simulink model "AHRS_Voter_Harness_HLR_13"  (R2025a)
settings: Solver=FixedStepDiscrete  StartTime=0.0  StopTime=10.0  RelTol=1e-3  EnableMultiTasking=on
Description:
  | Test harness for HLR_13.
settings Model: DataDictionary=DD_AHRS_Voter.sldd  EnableAccessToBaseWorkspace=off  Creator=The MathWorks, Inc.  LastModifiedBy=The MathWorks, Inc.
settings SolverCC: AlgebraicLoopSolver=TrustRegion  MaxZcPerStep=1.0
settings DataIOCC: LimitDataPoints=on
settings OptimizationCC: BlockReduction=off  DefaultParameterBehavior=Inlined  UseDivisionForNetSlopeComputation=on  UseFloatMulNetSlope=on  InlineInvariantSignals=on  EnhancedBackFolding=on  PassReuseOutputArgsAs=Individual arguments  EfficientFloat2IntCast=on  EfficientMapNaN2IntZero=off  LifeSpan=inf  MaxStackSize=inf  OptimizeBlockOrder=speed  EfficientTunableParamExpr=on
settings DebuggingCC: SignalInfNanChecking=error  SignalRangeChecking=error  ReadBeforeWriteMsg=EnableAllAsError  WriteAfterWriteMsg=EnableAllAsError  WriteAfterReadMsg=EnableAllAsError  AlgebraicLoopMsg=error  ArtificialAlgebraicLoopMsg=error  SaveWithDisabledLinksMsg=error  SaveWithParameterizedLinksMsg=error  BlockPriorityViolationMsg=error  SolverPrmCheckMsg=error  InheritedTsInSrcMsg=error  SingleTaskRateTransMsg=error  TasksWithSamePriorityMsg=error  SigSpecEnsureSampleTimeMsg=error  CheckMatrixSingularityMsg=error  IntegerOverflowMsg=error  ParameterUnderflowMsg=error  ParameterPrecisionLossMsg=error  ParameterTunabilityLossMsg=error  UnderSpecifiedDataTypeMsg=error  UnnecessaryDatatypeConvMsg=warning  VectorMatrixConversionMsg=error  SignalLabelMismatchMsg=error  UnconnectedInputMsg=error  UnconnectedOutputMsg=error  UnconnectedLineMsg=error  SFcnCompatibilityMsg=error  UniqueDataStoreMsg=error  BusObjectLabelMismatch=error  RootOutportRequireBusObject=error  AssertControl=DisableAll  AllowSymbolicDim=off  ModelReferenceIOMismatchMessage=error  UnknownTsInhSupMsg=error  ModelReferenceDataLoggingMessage=error  ModelReferenceSymbolNameMessage=none  StateNameClashWarn=warning  PregeneratedLibrarySubsystemCodeDiagnostic=none  StrictBusMsg=ErrorOnBusTreatedAsVector  NonBusSignalsTreatedAsBus=error  SFInvalidInputDataAccessInChartInitDiag=error  SFTransitionOutsideNaturalParentDiag=error  SFUnreachableExecutionPathDiag=error  SFUndirectedBroadcastEventsDiag=error  SFTransitionActionBeforeConditionDiag=error  SFExecutionAtInitializationDiag=none  IntegerSaturationMsg=error  ArithmeticOperatorsInVariantConditions=warning
settings HardwareCC: ProdBitPerPointer=32.0  ProdBitPerSizeT=32.0  ProdBitPerPtrDiffT=32.0  ProdLargestAtomicInteger=Long  ProdWordSize=32.0  ProdHWDeviceType=ARM Compatible->ARM 10
settings ModelReferenceCC: EnableRefExpFcnMdlSchedulingChecks=on  ModelReferenceNumInstancesAllowed=Single  PropagateSignalLabelsOutOfModel=off
settings SFSimCC: CompileTimeRecursionLimit=0.0  EnableRuntimeRecursion=off  MATLABDynamicMemAlloc=off  CustomCodeUndefinedFunction=UseInterfaceOnly
settings RTWCC: SystemTargetFile=ert.tlc  GenCodeOnly=on  TemplateMakefile=ert_default_tmf  GenerateReport=on  BuildConfiguration=Faster Runs  IncludeHyperlinkInReport=on  LaunchReport=on  GenerateTraceInfo=on  GenerateTraceReport=on  GenerateTraceReportSl=on  GenerateTraceReportSf=on  GenerateTraceReportEml=on  GenerateCodeMetricsReport=on  GPUComputeCapability=3.5  DLArmComputeVersion=19.05  Description=Embedded Coder
settings CodeAppCC: ForceParamTrailComments=on  IgnoreCustomStorageClasses=off  MATLABFcnDesc=on  MangleLength=4.0  StateflowObjectComments=on  ReqsInCode=on
settings ERTTargetCC: ExtModeTransport=0.0  ExtModeStaticAlloc=off  ExtModeMexFile=ext_comm  ExtModeIntrfLevel=Level1  ERTCustomFileTemplate=example_file_process.tlc  PreserveExpressionOrder=on  PreserveIfCondition=on  SuppressUnreachableDefaultCases=off  EnableSignedLeftShifts=off  EnableSignedRightShifts=off  DynamicArrayContainerType=coder::array  TargetLangStandard=C99 (ISO)  UtilityFuncGeneration=Shared location  GenerateSampleERTMain=on  IncludeMdlTerminateFcn=off  SuppressErrorStatus=on  SupportAbsoluteTime=off  SubcomponentCodeInterfacePackaging=Nonreusable function  SupportNonFinite=off  RemoveDisableFunc=on  ParenthesesLevel=Maximum  CastingMode=Standards  GenerateSharedConstants=off

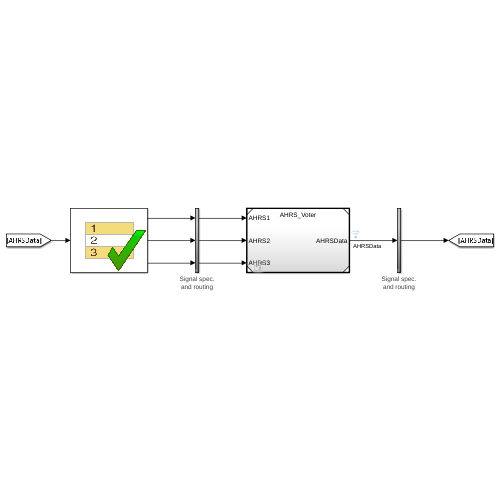
[thumbnail: Simulink's stored preview of the top-level diagram]
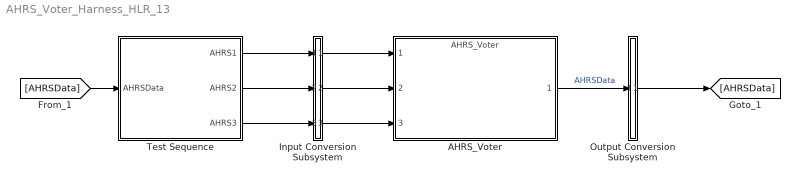
== system AHRS_Voter_Harness_HLR_13 ==
  AHRS_Voter : ModelReference  ModelNameDialog=AHRS_Voter  SimulationMode=Normal  ModelReferenceVersion=3.0
  Input Conversion Subsystem : Subsystem  Tag=__SLT_ICS__  Description=|
      | Signal spec.
      | and routing
      settings: AttributesFormatString=%<Description>
  Output Conversion Subsystem : Subsystem  Tag=__SLT_OCS__  Description=|
      | Signal spec.
      | and routing
      settings: AttributesFormatString=%<Description>
  Test Sequence : Test Sequence  TreatAsAtomicUnit=on
  wires:
  Test Sequence/1(AHRS1) -> Input Conversion Subsystem/1(Inport_1)
  Test Sequence/2(AHRS2) -> Input Conversion Subsystem/2(Inport_2)
  Test Sequence/3(AHRS3) -> Input Conversion Subsystem/3(Inport_3)
  [AHRSData] -> Test Sequence/1(AHRSData)
  Output Conversion Subsystem/1(Outport_1) -> [AHRSData]
  Input Conversion Subsystem/1(Outport_1) -> AHRS_Voter/1
  Input Conversion Subsystem/2(Outport_2) -> AHRS_Voter/2
  Input Conversion Subsystem/3(Outport_3) -> AHRS_Voter/3
  AHRS_Voter/1 -> Output Conversion Subsystem/1(Inport_1)  "AHRSData"

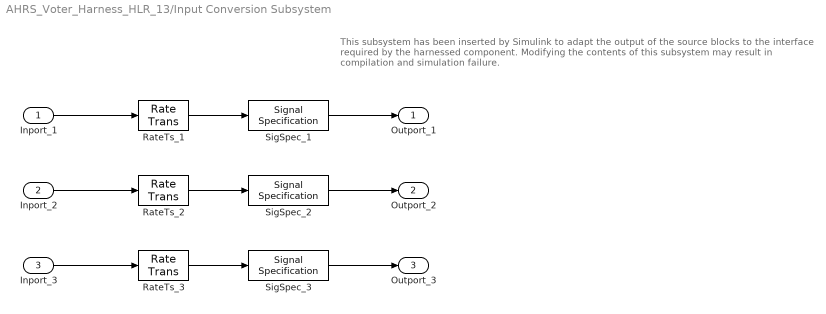
== system AHRS_Voter_Harness_HLR_13/Input Conversion Subsystem ==
  note: This subsystem has been inserted by Simulink to adapt the output of the source blocks to the interface required by the harnessed component.
      |  Modifying the contents of this subsystem may result in compilation and simulation failure.
  Inport_1 : Inport
  Inport_2 : Inport  Port=2
  Inport_3 : Inport  Port=3
  RateTs_1 : RateTransition  OutPortSampleTime=0.01
  RateTs_2 : RateTransition  OutPortSampleTime=0.01
  RateTs_3 : RateTransition  OutPortSampleTime=0.01
  SigSpec_1 : SignalSpecification  OutDataTypeStr=Bus: AHRS_Bus  Dimensions=[1]  SampleTime=0.01  BusOutputAsStruct=on
  SigSpec_2 : SignalSpecification  OutDataTypeStr=Bus: AHRS_Bus  Dimensions=[1]  SampleTime=0.01  BusOutputAsStruct=on
  SigSpec_3 : SignalSpecification  OutDataTypeStr=Bus: AHRS_Bus  Dimensions=[1]  SampleTime=0.01  BusOutputAsStruct=on
  Outport_1 : Outport  VectorParamsAs1DForOutWhenUnconnected=off
  Outport_2 : Outport  Port=2  VectorParamsAs1DForOutWhenUnconnected=off
  Outport_3 : Outport  Port=3  VectorParamsAs1DForOutWhenUnconnected=off
  wires:
  SigSpec_1/1 -> Outport_1/1
  RateTs_1/1 -> SigSpec_1/1
  Inport_1/1 -> RateTs_1/1
  SigSpec_2/1 -> Outport_2/1
  RateTs_2/1 -> SigSpec_2/1
  Inport_2/1 -> RateTs_2/1
  SigSpec_3/1 -> Outport_3/1
  RateTs_3/1 -> SigSpec_3/1
  Inport_3/1 -> RateTs_3/1

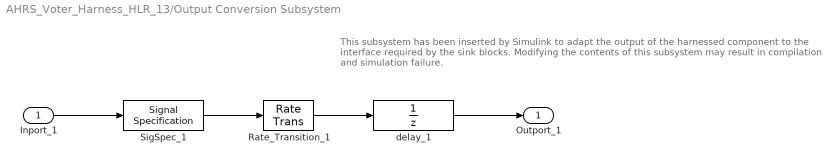
== system AHRS_Voter_Harness_HLR_13/Output Conversion Subsystem ==
  note: This subsystem has been inserted by Simulink to adapt the output of the harnessed component to the interface required by the sink blocks.
      |  Modifying the contents of this subsystem may result in compilation and simulation failure.
  Inport_1 : Inport
  Rate_Transition_1 : RateTransition  OutPortSampleTimeOpt=Inherit
  SigSpec_1 : SignalSpecification  OutDataTypeStr=double  Dimensions=[5]  SampleTime=0.01
  delay_1 : UnitDelay  SampleTime=-1  HasFrameUpgradeWarning=on
  Outport_1 : Outport  VectorParamsAs1DForOutWhenUnconnected=off
  wires:
  Inport_1/1 -> SigSpec_1/1
  SigSpec_1/1 -> Rate_Transition_1/1
  Rate_Transition_1/1 -> delay_1/1
  delay_1/1 -> Outport_1/1

== stateflow chart AHRS_Voter_Harness_HLR_13/Test Sequence ==
  state step_0
    %% Initialize data outputs.
    AHRS1.valid = true;
    AHRS1.theta = 0;
    AHRS1.phi = 0;
    AHRS1.r = 0;
    AHRS1.q = 0;
    AHRS1.p = 0;
    AHRS2.valid = true;
    AHRS2.theta = 0;
    AHRS2.phi = 0;
    AHRS2.r = 0;
    AHRS2.q = 0;
    AHRS2.p = 0;
    AHRS3.valid = true;
    AHRS3.theta = 0;
    AHRS3.phi = 0;
    AHRS3.r = 0;
    AHRS3.q = 0;
    AHRS3.p = 0;
  state step_1
    % Test that all outputs are set to zero uisng the tolerance
    verify(abs(AHRSData(1))<Tol, 'HLR13 step_1: Zero output condition failed for theta');
    verify(abs(AHRSData(2))<Tol, 'HLR13 step_1: Zero output condition failed for phi');
    verify(abs(AHRSData(3))<Tol, 'HLR13 step_1: Zero output condition failed for r');
    verify(abs(AHRSData(4))<Tol, 'HLR13 step_1: Zero output condition failed for q');
    verify(abs(AHRSData(5))<Tol, 'HLR13 step_1: Zero output condition failed for p');
  state step_2
    % Set each AHRS to have different data and only AHRS 1 to valid.
    % AHRS1
    AHRS1.valid = true;
    AHRS1.theta = 1;
    AHRS1.phi = 1;
    AHRS1.r = 1;
    AHRS1.q = 1;
    AHRS1.p = 1;
    % AHRS2
    AHRS2.valid = false;
    AHRS2.theta = 0;
    AHRS2.phi = 0;
    AHRS2.r = 0;
    AHRS2.q = 0;
    AHRS2.p = 0;
    % AHRS3
    AHRS3.valid = false;
    AHRS3.theta = -1;
    AHRS3.phi = -1;
    AHRS3.r = -1;
    AHRS3.q = -1;
    AHRS3.p = -1;
  state step_3
    % Test that each signal is using AHRS1 data, psi is unused
    verify(abs(AHRSData(1)-AHRS1.theta)<Tol, ' HLR_13 step_3: AHRS1 theta selection failed');
    verify(abs(AHRSData(2)-AHRS1.phi)<Tol, ' HLR_13 step_3: AHRS1 phi selection failed');
    verify(abs(AHRSData(3)-AHRS1.r)<Tol, ' HLR_13 step_3: AHRS1 r selection failed');
    verify(abs(AHRSData(4)-AHRS1.q)<Tol, ' HLR_13 step_3: AHRS1 q  selection failed');
    verify(abs(AHRSData(5)-AHRS1.p)<Tol, ' HLR_13 step_3: AHRS1 p selection failed');
  state step_4
    % Set only AHRS2 to valid
    AHRS1.valid = false;
    AHRS2.valid = true;
  state step_5
    % Test that each signal is using AHRS2 data, psi is unused
    verify(abs(AHRSData(1)-AHRS2.theta)<Tol, 'HLR_13 step_5: AHRS2 theta selection failed');
    verify(abs(AHRSData(2)-AHRS2.phi)<Tol, 'HLR_13 step_5: AHRS2 phi selection failed');
    verify(abs(AHRSData(3)-AHRS2.r)<Tol, 'HLR_13 step_5: AHRS2 r selection failed');
    verify(abs(AHRSData(4)-AHRS2.q)<Tol, 'HLR_13 step_5: AHRS2 q selection failed');
    verify(abs(AHRSData(5)-AHRS2.p)<Tol, 'HLR_13 step_5: AHRS2 p selection failed');
  state step_6
    % Set only AHRS3 to valid
    AHRS2.valid = false;
    AHRS3.valid = true;
  state step_7
    % Test that each signal is using AHRS3 data, psi is unused
    verify(abs(AHRSData(1)-AHRS3.theta)<Tol, 'HLR_13 step_7: AHRS3 theta selection failed');
    verify(abs(AHRSData(2)-AHRS3.phi)<Tol, 'HLR_13 step_7: AHRS3 phi selection failed');
    verify(abs(AHRSData(3)-AHRS3.r)<Tol, 'HLR_13 step_7: AHRS3 r selection failed');
    verify(abs(AHRSData(4)-AHRS3.q)<Tol, 'HLR_13 step_7: AHRS3 q selection failed');
    verify(abs(AHRSData(5)-AHRS3.p)<Tol, 'HLR_13 step_7: AHRS3 p selection failed');
  (default) -> step_0
  step_0 -> step_1 : [after(1, sec)
      | ]
  step_1 -> step_2
  step_2 -> step_3 : [after(1, sec)
      | ]
  step_3 -> step_4
  step_4 -> step_5 : [after(1, sec)
      | ]
  step_5 -> step_6
  step_6 -> step_7 : [after(1, sec)
      | ]
  data: AHRSData input double size=[5]; AHRS1 output Bus: AHRS_Bus size=[1]; AHRS2 output Bus: AHRS_Bus size=[1]; AHRS3 output Bus: AHRS_Bus size=[1]; Tol constant double =1e-7
